simulink model "psb3phlinereclose"  (Simulink 6.0)
settings: Solver=FixedStepDiscrete  StartTime=0.0  StopTime=0.7  FixedStep=50e-6  RelTol=1e-4
InitFcn:
  | powericon('psbinitsys',bdroot);
undefined symbols (not defined in the file or in its folder): D1, Delta, rvar
libraries: powerlib2 x33, powerlib_extras x2
settings Model: Creator=sybille  LastModifiedBy=batserve  ExtModeTrigMode=oneshot  ExtModeArmWhenConnect=off  ExtModeAutoUpdateStatusClock=off
settings DataIOCC: LimitDataPoints=off  SignalLoggingName=sigsOut
settings OptimizationCC: BlockReduction=off  BooleanDataType=off
settings DebuggingCC: CheckExecutionContextPreStartOutputMsg=on  CheckExecutionContextRuntimeOutputMsg=on  SolverPrmCheckMsg=none
settings HardwareCC: TargetUnknown=on

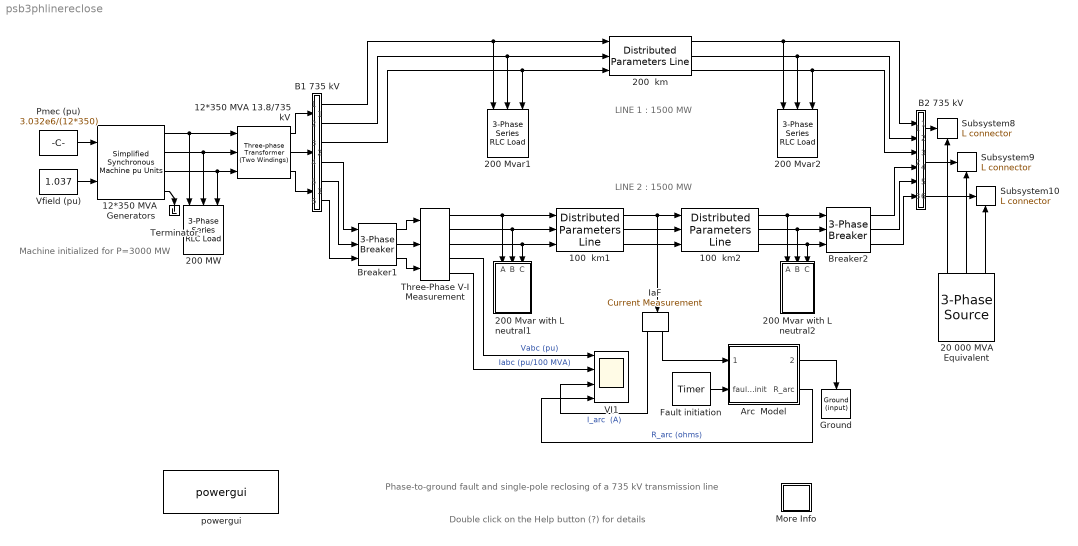
== system psb3phlinereclose ==
  note: Machine initialized
      |  for P=3000 MW
  note: Phase-to-ground fault and single-pole reclosing
      | of  a 735 kV transmission line
  note: Double click on the Help button (?) for details
  note: LINE 1 : 1500 MW
  note: LINE 2 : 1500 MW
  " Breaker1" : powerlib2/Elements/3-Phase Breaker  init_states=closed  sa=on  sb=off  sc=off  sw_times="[4/60  34/60]"  Ts=50e-6  comext=off  Ron=0.001  Rp=1e5  Cp=inf  mesure=None
  " Breaker2" : powerlib2/Elements/3-Phase Breaker  init_states=closed  sa=on  sb=off  sc=off  sw_times="[4/60  34/60]"  Ts=50e-6  comext=off  Ron=0.001  Rp=1e5  Cp=inf  mesure=None
  100  km1 : powerlib2/Elements/Distributed Parameters Line  Tag=PoWeRsYsTeMbLoCk  n=3  f=60  r=[0.01165 0.2676]  l="[0.8679e-3  3.008e-3]"  c="[13.41e-9  8.57e-9]"  lgt=100  x1=[0 -2.416e-007 4.728e+005 -5.555e+005;0.0001015 -2.421e-007 4.937e+005 -5.37e+005;0.0002031 -2.424e-007 5.139e+005 -5.177e+005;0.0003046 -2.422e-007 5.333e+005 -4.977e+005;0.0004062 -2.417e-007 5.52e+005 -4.769e+005;0.0005077 -2.408e-007 5.699e+005 -4.554e+005]  x2=[0 -1.471e-007 4.261e+005 -5.969e+005;0.0001015 -1.474e-007 4.486e+005 -5.801e+005;0.0002031 -1.474e-007 4.705e+005 -5.625e+005;0.0003046 -1.472e-007 4.917e+005 -5.441e+005;0.0004062 -1.468e-007 5.122e+005 -5.249e+005;0.0005077 -1.462e-007 5.319e+005 -5.049e+005]  x3=[0 -2.944e-010 398.8 -914.4;0.0001015 -2.663e-010 433.5 -898.5;0.0002031 -2.378e-010 467.6 -881.2;0.0003046 -2.089e-010 501 -862.7;0.0004062 -1.797e-010 533.6 -842.9;0.0005077 -1.503e-010 565.5 -821.9]  x4=[0 -3.362e-010 2831 -3827;0.0001015 -3.679e-010 2976 -3716;0.0002031 -3.99e-010 3116 -3599;0.0003046 -4.295e-010 3251 -3477;0.0004062 -4.594e-010 3382 -3350;0.0005077 -4.886e-010 3508 -3218]  x5=0.0005077  mesure=None  PSBOutputType=111111111111111111111111111111
  100  km2 : powerlib2/Elements/Distributed Parameters Line  Tag=PoWeRsYsTeMbLoCk  n=3  f=60  r=[0.01165 0.2676]  l="[0.8679e-3  3.008e-3]"  c="[13.41e-9  8.57e-9]"  lgt=100  x1=[0 -1.471e-007 4.261e+005 -5.969e+005;0.0001015 -1.474e-007 4.486e+005 -5.801e+005;0.0002031 -1.474e-007 4.705e+005 -5.625e+005;0.0003046 -1.472e-007 4.917e+005 -5.441e+005;0.0004062 -1.468e-007 5.122e+005 -5.249e+005;0.0005077 -1.462e-007 5.319e+005 -5.049e+005]  x2=[0 -4.673e-008 3.727e+005 -6.281e+005;0.0001015 -4.666e-008 3.965e+005 -6.134e+005;0.0002031 -4.652e-008 4.197e+005 -5.978e+005;0.0003046 -4.631e-008 4.422e+005 -5.813e+005;0.0004062 -4.604e-008 4.642e+005 -5.639e+005;0.0005077 -4.569e-008 4.854e+005 -5.457e+005]  x3=[0 -1.263e-010 506.9 -849.4;0.0001015 -9.531e-011 539.1 -829.3;0.0002031 -6.416e-011 570.4 -808.1;0.0003046 -3.291e-011 600.9 -785.7;0.0004062 -1.62e-012 630.6 -762.1;0.0005077 2.968e-011 659.3 -737.4]  x4=[0 -1.89e-010 2313 -4151;0.0001015 -2.214e-010 2470 -4059;0.0002031 -2.535e-010 2624 -3962;0.0003046 -2.852e-010 2773 -3859;0.0004062 -3.164e-010 2919 -3750;0.0005077 -3.472e-010 3060 -3635]  x5=0.0005077  mesure=None  PSBOutputType=111111111111111111111111111111
  12*350 MVA 13.8/735 kV : powerlib2/Elements/Three-phase Transformer (Two Windings)  Tag=PoWeRsYsTeMbLoCk  nominal=[ 12*350e6 , 60 ]  type1=Delta (D1)  params1=[ 13.8e3 , 0.002 , 0.08 ]  type2=Yg  params2=[ 735e3 , 0.002 , 0.08 ]  ynsat=off  rmag=500  lm=500  sat=[ 0,0 ; 0.0024,1.2 ; 1.0,1.52 ]  hyst=off  matfile='hysteresis'  sif=off  phi0=[ 0.8 , -0.8 , 0.7 ]  initialslopes=[+1 +1 +1]  mesure=None  PSBOutputType=111
  12*350 MVA  Generators : powerlib2/Machines/Simplified Synchronous  Machine  pu Units  Tag=PoWeRsYsTeMbLoCk  conType=3-wire Y  x1=[ 12*350e6,13.8e3,60 ]  x2=[ inf,0,2 ]  x3=[ 0.22/15, 0.22 ]  x4=[0 2.57573 0.717405 0.717405 0.717405 -11.4304 -131.43 108.57]  PSBOutputType=1110  iounits=0  LoadFlowParameters=[1 3000000000 0 0 0]
  20 000 MVA Equivalent : powerlib2/Electrical Sources/3-Phase Source  Tag=PoWeRsYsTeMbLoCk  Orientation=up  V=735e3  Phi=0  F=60  InternalConnection=Yg  RLoff=on  R=735^2/20000/10  L=735^2/20000/377  Psc=20000e6  Vbase=735e3  XRratio=10  PSBOutputType=111
  200  km : powerlib2/Elements/Distributed Parameters Line  Tag=PoWeRsYsTeMbLoCk  n=3  f=60  r=[0.01165 0.2676]  l="[0.8679e-3  3.008e-3]"  c="[13.41e-9  8.57e-9]"  lgt=200  x1=[0 -2.332e-007 3.976e+005 -6.116e+005;0.0002031 -2.374e-007 4.433e+005 -5.794e+005;0.0004062 -2.403e-007 4.863e+005 -5.438e+005;0.0006093 -2.417e-007 5.264e+005 -5.05e+005;0.0008124 -2.417e-007 5.635e+005 -4.632e+005;0.001015 -2.403e-007 5.973e+005 -4.188e+005]  x2=[0 -4.613e-008 2.891e+005 -6.707e+005;0.0002031 -4.657e-008 3.395e+005 -6.466e+005;0.0004062 -4.675e-008 3.88e+005 -6.188e+005;0.0006093 -4.665e-008 4.342e+005 -5.873e+005;0.0008124 -4.628e-008 4.779e+005 -5.524e+005;0.001015 -4.563e-008 5.187e+005 -5.142e+005]  x3=[0 -4.038e-010 276 -953;0.0002031 -3.531e-010 348.1 -929.1;0.0004062 -3.004e-010 418.1 -899.7;0.0006093 -2.46e-010 485.7 -865.1;0.0008124 -1.901e-010 550.5 -825.4;0.001015 -1.331e-010 612 -780.9]  x4=[0 -1.229e-011 1756 -4400;0.0002031 -7.699e-011 2087 -4253;0.0004062 -1.412e-010 2407 -4081;0.0006093 -2.046e-010 2712 -3885;0.0008124 -2.669e-010 3001 -3666;0.001015 -3.275e-010 3273 -3426]  x5=0.001015  mesure=None  PSBOutputType=111111111111111111111111111111
  200 MW : powerlib2/Elements/3-Phase Series RLC Load  Orientation=down  Vpp=13.8e3  fn=60  P3=200e6  QL3=0  QC3=0
  200 Mvar with L neutral1 : Subsystem  Orientation=down
  200 Mvar with L neutral2 : Subsystem  Orientation=down
  200 Mvar1 : powerlib2/Elements/3-Phase Series RLC Load  Orientation=down  Vpp=735e3  fn=60  P3=200e6/250  QL3=200e6  QC3=0
  200 Mvar2 : powerlib2/Elements/3-Phase Series RLC Load  Orientation=down  Vpp=735e3  fn=60  P3=200e6/250  QL3=200e6  QC3=0
  Arc  Model : Subsystem  mask(Arc model){Rarc_var=on, Rarc_fixed=0.1, Rparam=[56.54 0.006375], I0=50, Ts=50e-6}
      mask prompts: Rarc_var "Variable arc resistance :"; Rarc_fixed "Arc resistance for fixed arc resistance :"; Rparam "Arc parameters for variable arc resistance [Ro k] : :"; I0 "Current threshold for arc extinction Io (A rms) :"; Ts "Sample time (s) :"
      mask help:
      | This block implements a variable or fixed arc resistance model.
      |
      | Input 1, output 1:  Connection terminals of the arc
      |                              resistance.
      | Input 2 :    Control signal for the fault initiation
      | Use a short pulse of 1 cycle. Once fault current starts flowing, it is sustained by the arc ionized path.
      | Output 2:  Arc resitance
      |
      | If you check the 'Variable arc resistance' box, the mean arc resistance will be a function of the arc current, according to equation. Otherwise, the resistance will be kept constant.
      |
      |        Rarc= Ro*exp(-k*i)
      |
      | where:   i = rms value of the arc current (A)
      |              Ro, k = arc parameters
      |
      | The arc extinguishes at the next zero current crossing after its  rms value has fallen  below  the specified threshold current Io.
      mask init:
      | if strcmp(Rarc_var,'on'), rvar=1; else, rvar=0; end
      | R0=Rparam(1);
      | k=Rparam(2);
  B1 735 kV : Subsystem
      mask Display: disp('')
  B2 735 kV : Subsystem
      mask Display: disp('')
  Fault initiation : powerlib_extras/Control  Blocks/Timer  t=[ 1/60 2/60 ]  e="[1 0  ]"
  Ground : powerlib2/Connectors/Ground (input)  Tag=PoWeRsYsTeMbLoCk  Orientation=down
  IaF : powerlib2/Measurements/Current Measurement  Tag=PoWeRsYsTeMmEaSuReMeNt  Orientation=down  PhasorSimulation=off  OutputType=Magnitude  PSBOutputType=01  PSBequivalent=0
  More Info : Subsystem
      mask Display: disp('?')
  Pmec (pu) : Constant  Value=3.032e6/(12*350)
  Subsystem10 : powerlib2/Connectors/L connector  Tag=PoWeRsYsTeMbLoCk  Orientation=up
  Subsystem8 : powerlib2/Connectors/L connector  Tag=PoWeRsYsTeMbLoCk  Orientation=up
  Subsystem9 : powerlib2/Connectors/L connector  Tag=PoWeRsYsTeMbLoCk  Orientation=up
  Terminator : Terminator
      settings: Orientation=down
  Three-Phase V-I Measurement : powerlib2/Measurements/Three-Phase V-I Measurement  Tag=PoWeRsYsTeMmEaSuReMeNt  VChoice=phase-to-ground  ualv=off  labelV=V1  Vpu=on  Vbase=735e3  IChoice=yes  ualc=off  labelC=I1  Ppu=on  Pbase=100e6  OutputType=Magnitude  PhasorSimulation=off  PSBequivalent=1  PSBOutputType=11100
  VI1 : Scope  NumInputPorts=4
      settings: TimeRange=0.7000000000000001  YMin=-2~-100~-50000~0  YMax=2~100~50000~100  DataFormat=Array
  Vfield (pu) : Constant  Value=1.037
  powergui : powerlib2/powergui  Frange=logspace(0,3,50)  Ylog=off  Xlog=off  save=off  variable=ZData  ZoomFFT=on  StartTime=0.0  cycles=1  DisplayStyle=off  fundamental=60  FreqAxis=off  MaxFrequency=1000  frequencyindice=60  frequencyindicesteady=1  RmsSteady=1  display=off  Ts=50e-6  methode=off  frequency=60  echomessages=off
  wires:
  " Breaker1"/1 -> Three-Phase V-I Measurement/1
  " Breaker1"/2 -> Three-Phase V-I Measurement/2
  " Breaker1"/3 -> Three-Phase V-I Measurement/3
  12*350 MVA 13.8/735 kV/1 -> B1 735 kV/1(A1)
  12*350 MVA 13.8/735 kV/2 -> B1 735 kV/2(B1)
  12*350 MVA 13.8/735 kV/3 -> B1 735 kV/3(C1)
  B1 735 kV/4(A4) -> " Breaker1"/1
  B1 735 kV/5(B4) -> " Breaker1"/2
  B1 735 kV/6(C4) -> " Breaker1"/3
  12*350 MVA  Generators/1 -> 12*350 MVA 13.8/735 kV/1, 200 MW/1
  12*350 MVA  Generators/2 -> 12*350 MVA 13.8/735 kV/2, 200 MW/2
  12*350 MVA  Generators/3 -> 12*350 MVA 13.8/735 kV/3, 200 MW/3
  Vfield (pu)/1 -> 12*350 MVA  Generators/2
  Pmec (pu)/1 -> 12*350 MVA  Generators/1
  " Breaker2"/3 -> B2 735 kV/6(C2)
  B2 735 kV/1(A3) -> Subsystem8/Enable
  20 000 MVA Equivalent/1 -> Subsystem8/1
  B2 735 kV/2(B3) -> Subsystem9/Enable
  20 000 MVA Equivalent/2 -> Subsystem9/1
  B2 735 kV/3(C3) -> Subsystem10/Enable
  20 000 MVA Equivalent/3 -> Subsystem10/1
  " Breaker2"/1 -> B2 735 kV/4(A2)
  " Breaker2"/2 -> B2 735 kV/5(B2)
  100  km2/1 -> " Breaker2"/1, 200 Mvar with L neutral2/1(A)
  100  km2/2 -> " Breaker2"/2, 200 Mvar with L neutral2/2(B)
  100  km2/3 -> " Breaker2"/3, 200 Mvar with L neutral2/3(C)
  100  km1/1 -> 100  km2/1, IaF/1
  B1 735 kV/1(A3) -> 200  km/1, 200 Mvar1/1
  B1 735 kV/2(B3) -> 200  km/2, 200 Mvar1/2
  B1 735 kV/3(C3) -> 200  km/3, 200 Mvar1/3
  200  km/1 -> B2 735 kV/1(A1`), 200 Mvar2/1
  200  km/2 -> B2 735 kV/2(B1), 200 Mvar2/2
  200  km/3 -> B2 735 kV/3(C1), 200 Mvar2/3
  Three-Phase V-I Measurement/1 -> 100  km1/1, 200 Mvar with L neutral1/1(A)
  Three-Phase V-I Measurement/2 -> 100  km1/2, 200 Mvar with L neutral1/2(B)
  Three-Phase V-I Measurement/3 -> 100  km1/3, 200 Mvar with L neutral1/3(C)
  100  km1/3 -> 100  km2/3
  100  km1/2 -> 100  km2/2
  Three-Phase V-I Measurement/4 -> VI1/1  "Vabc (pu)"
  Fault initiation/1 -> Arc  Model/2(fault_init)
  Arc  Model/1(2) -> Ground/1
  IaF/2 -> Arc  Model/1(1)
  IaF/1 -> VI1/3  "I_arc  (A)"
  Arc  Model/2(R_arc) -> VI1/4  "R_arc (ohms)"
  Three-Phase V-I Measurement/5 -> VI1/2  "Iabc (pu/100 MVA)"
  12*350 MVA  Generators/4 -> Terminator/1

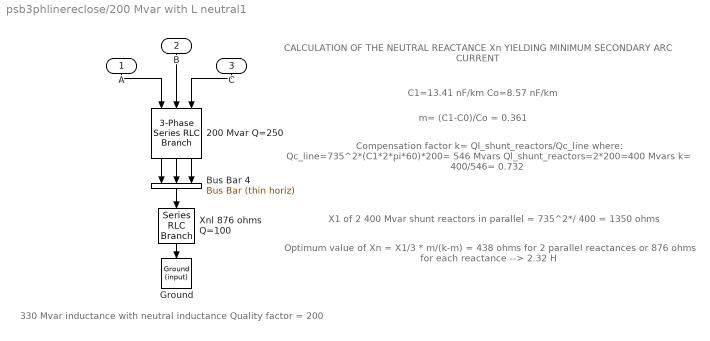
== system psb3phlinereclose/200 Mvar with L neutral1 ==
  note: CALCULATION OF THE NEUTRAL REACTANCE Xn
      | YIELDING MINIMUM SECONDARY ARC CURRENT
  note: X1 of 2 400 Mvar shunt reactors in parallel = 735^2*/ 400 = 1350 ohms
  note: Optimum value of Xn = X1/3 * m/(k-m) = 438 ohms for 2 parallel reactances
      | or 876 ohms for each reactance --> 2.32 H
  note: Compensation factor k= Ql_shunt_reactors/Qc_line
      | where:
      |  Qc_line=735^2*(C1*2*pi*60)*200= 546 Mvars
      |  Ql_shunt_reactors=2*200=400 Mvars
      | k= 400/546= 0.732
  note: m= (C1-C0)/Co = 0.361
  note: C1=13.41 nF/km Co=8.57 nF/km
  note: 330 Mvar inductance
      | with neutral inductance
      | Quality factor = 200
  A : Inport  Orientation=down  Port=1  LatchInput=off
  B : Inport  Orientation=down  Port=2  LatchInput=off
  C : Inport  Orientation=down  Port=3  LatchInput=off
  200 Mvar Q=250 : powerlib2/Elements/3-Phase Series RLC Branch   Orientation=down  R=735^2/200/250  L=735^2/200/377  C=inf
  Bus Bar 4 : powerlib2/Connectors/Bus Bar (thin horiz)  Tag=PoWeRsYsTeMbLoCk  Orientation=down  input=3  output=1  PSBOutputType=111111111111111111111111111111111111111111111111111111111111111111111111111111111111
  Ground : powerlib2/Connectors/Ground (input)  Tag=PoWeRsYsTeMbLoCk  Orientation=down
  Xnl 876 ohms Q=100 : powerlib2/Elements/Series RLC Branch  Tag=PoWeRsYsTeMbLoCk  Orientation=down  a=876/100  b=876/377  c=inf  mesure=None  PSBOutputType=1
  wires:
  A/1 -> 200 Mvar Q=250/1
  B/1 -> 200 Mvar Q=250/2
  C/1 -> 200 Mvar Q=250/3
  200 Mvar Q=250/1 -> Bus Bar 4/1
  200 Mvar Q=250/3 -> Bus Bar 4/3
  200 Mvar Q=250/2 -> Bus Bar 4/2
  Bus Bar 4/1 -> Xnl 876 ohms Q=100/1
  Xnl 876 ohms Q=100/1 -> Ground/1

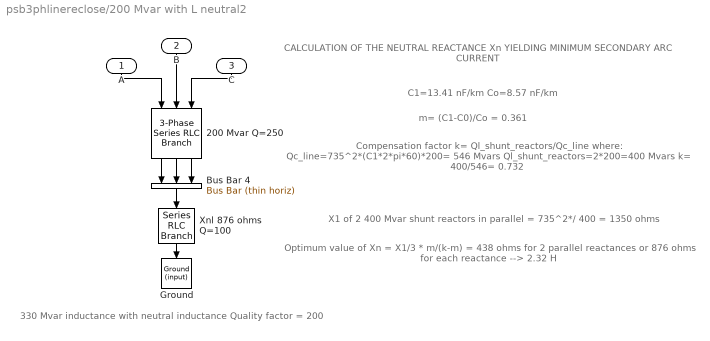
== system psb3phlinereclose/200 Mvar with L neutral2 ==
  note: 330 Mvar inductance
      | with neutral inductance
      | Quality factor = 200
  note: C1=13.41 nF/km Co=8.57 nF/km
  note: m= (C1-C0)/Co = 0.361
  note: Compensation factor k= Ql_shunt_reactors/Qc_line
      | where:
      |  Qc_line=735^2*(C1*2*pi*60)*200= 546 Mvars
      |  Ql_shunt_reactors=2*200=400 Mvars
      | k= 400/546= 0.732
  note: Optimum value of Xn = X1/3 * m/(k-m) = 438 ohms for 2 parallel reactances
      | or 876 ohms for each reactance --> 2.32 H
  note: X1 of 2 400 Mvar shunt reactors in parallel = 735^2*/ 400 = 1350 ohms
  note: CALCULATION OF THE NEUTRAL REACTANCE Xn
      | YIELDING MINIMUM SECONDARY ARC CURRENT
  A : Inport  Orientation=down  Port=1  LatchInput=off
  B : Inport  Orientation=down  Port=2  LatchInput=off
  C : Inport  Orientation=down  Port=3  LatchInput=off
  200 Mvar Q=250 : powerlib2/Elements/3-Phase Series RLC Branch   Orientation=down  R=735^2/200/250  L=735^2/200/377  C=inf
  Bus Bar 4 : powerlib2/Connectors/Bus Bar (thin horiz)  Tag=PoWeRsYsTeMbLoCk  Orientation=down  input=3  output=1  PSBOutputType=111111111111111111111111111111111111111111111111111111111111111111111111111111111111
  Ground : powerlib2/Connectors/Ground (input)  Tag=PoWeRsYsTeMbLoCk  Orientation=down
  Xnl 876 ohms Q=100 : powerlib2/Elements/Series RLC Branch  Tag=PoWeRsYsTeMbLoCk  Orientation=down  a=876/100  b=876/377  c=inf  mesure=None  PSBOutputType=1
  wires:
  Xnl 876 ohms Q=100/1 -> Ground/1
  Bus Bar 4/1 -> Xnl 876 ohms Q=100/1
  200 Mvar Q=250/2 -> Bus Bar 4/2
  200 Mvar Q=250/3 -> Bus Bar 4/3
  200 Mvar Q=250/1 -> Bus Bar 4/1
  C/1 -> 200 Mvar Q=250/3
  B/1 -> 200 Mvar Q=250/2
  A/1 -> 200 Mvar Q=250/1

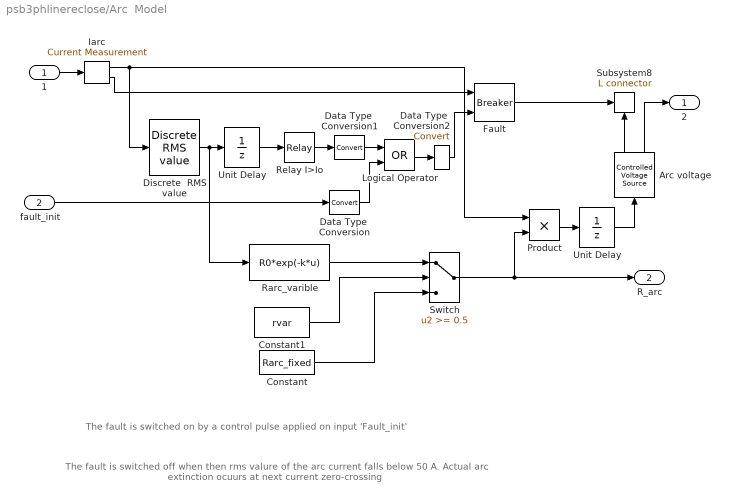
== system psb3phlinereclose/Arc  Model ==
  note: The fault is switched on by a control pulse applied on input 'Fault_init'
  note: The fault is switched off when then rms valure of the arc current falls below  50 A.
      | Actual arc extinction ocuurs at next current zero-crossing
  1 : Inport  Port=1  LatchInput=off
  fault_init : Inport  Port=2  LatchInput=off
  Arc voltage : powerlib2/Electrical Sources/Controlled Voltage Source  Tag=PoWeRsYsTeMbLoCk  Description=source block  Orientation=up  initsrc=on  srctyp=AC  iv=0  iph=0  ifreq=0  mesure=None  PSBOutputType=11
  Constant : Constant  Value=Rarc_fixed
  Constant1 : Constant  Value=rvar
  Data Type  Conversion : DataTypeConversion  OutDataTypeMode=boolean  SaturateOnIntegerOverflow=on  RndMeth=Zero
  Data Type  Conversion1 : DataTypeConversion  OutDataTypeMode=boolean  SaturateOnIntegerOverflow=on  RndMeth=Zero
  Data Type  Conversion2 : DataTypeConversion  OutDataTypeMode=double  SaturateOnIntegerOverflow=on  RndMeth=Zero
  Discrete  RMS value : powerlib_extras/Discrete Measurements/Discrete  RMS value  Freq=60  Mag_Init=0  Ts=Ts
  Fault : powerlib2/Elements/Breaker  Tag=PoWeRsYsTeMbLoCk  a=.001  c=0  rs=inf  cs=0  times="[ 4/60  5/60 ]"  Ts=0  comext=on  mesure=None  PSBOutputType=1
  Iarc : powerlib2/Measurements/Current Measurement  Tag=PoWeRsYsTeMmEaSuReMeNt  PhasorSimulation=off  OutputType=Magnitude  PSBOutputType=01  PSBequivalent=0
  Logical Operator : Logic  Operator=OR
  Product : Product  SaturateOnIntegerOverflow=on  InputSameDT=on
  Rarc_varible : Fcn  Expr=R0*exp(-k*u)
  Relay I>Io : Relay  OnSwitchValue=I0*1.2  OffSwitchValue=I0  ZeroCross=off
  Subsystem8 : powerlib2/Connectors/L connector  Tag=PoWeRsYsTeMbLoCk  Orientation=up
  Switch : Switch  Threshold=0.5  ZeroCross=off  InputSameDT=on
  Unit Delay : UnitDelay  SampleTime=Ts
  "Unit Delay " : UnitDelay  SampleTime=Ts
  2 : Outport
  R_arc : Outport  Port=2
  wires:
  1/1 -> Iarc/1
  Fault/1 -> Subsystem8/Enable
  Iarc/2 -> Fault/1
  Iarc/1 -> Discrete  RMS value/1, Product/1
  Discrete  RMS value/1 -> "Unit Delay "/1, Rarc_varible/1
  Rarc_varible/1 -> Switch/1
  Switch/1 -> Product/2, R_arc/1
  Constant/1 -> Switch/3
  Constant1/1 -> Switch/2
  Arc voltage/1 -> Subsystem8/1
  Arc voltage/2 -> 2/1
  Product/1 -> Unit Delay/1
  Unit Delay/1 -> Arc voltage/1
  "Unit Delay "/1 -> Relay I>Io/1
  fault_init/1 -> Data Type  Conversion/1
  Data Type  Conversion/1 -> Logical Operator/2
  Relay I>Io/1 -> Data Type  Conversion1/1
  Data Type  Conversion1/1 -> Logical Operator/1
  Logical Operator/1 -> Data Type  Conversion2/1
  Data Type  Conversion2/1 -> Fault/2

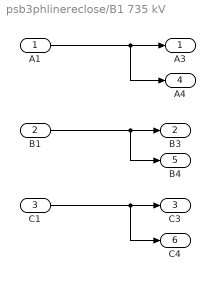
== system psb3phlinereclose/B1 735 kV ==
  A1 : Inport  Port=1  LatchInput=off
  B1 : Inport  Port=2  LatchInput=off
  C1 : Inport  Port=3  LatchInput=off
  A3 : Outport  InitialOutput=0
  B3 : Outport  Port=2  InitialOutput=0
  C3 : Outport  Port=3  InitialOutput=0
  A4 : Outport  Port=4  InitialOutput=0
  B4 : Outport  Port=5  InitialOutput=0
  C4 : Outport  Port=6  InitialOutput=0
  wires:
  C1/1 -> C3/1, C4/1
  B1/1 -> B3/1, B4/1
  A1/1 -> A3/1, A4/1

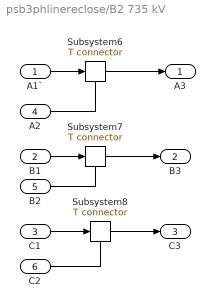
== system psb3phlinereclose/B2 735 kV ==
  A1` : Inport  Port=1  LatchInput=off
  B1 : Inport  Port=2  LatchInput=off
  C1 : Inport  Port=3  LatchInput=off
  A2 : Inport  Port=4  LatchInput=off
  B2 : Inport  Port=5  LatchInput=off
  C2 : Inport  Port=6  LatchInput=off
  Subsystem6 : powerlib2/Connectors/T connector  Tag=PoWeRsYsTeMbLoCk  PSBOutputType=1
  Subsystem7 : powerlib2/Connectors/T connector  Tag=PoWeRsYsTeMbLoCk  PSBOutputType=1
  Subsystem8 : powerlib2/Connectors/T connector  Tag=PoWeRsYsTeMbLoCk  PSBOutputType=1
  A3 : Outport  InitialOutput=0
  B3 : Outport  Port=2  InitialOutput=0
  C3 : Outport  Port=3  InitialOutput=0
  wires:
  C2/1 -> Subsystem8/Enable
  A2/1 -> Subsystem6/Enable
  B2/1 -> Subsystem7/Enable
  B1/1 -> Subsystem7/1
  C1/1 -> Subsystem8/1
  A1`/1 -> Subsystem6/1
  Subsystem8/1 -> C3/1
  Subsystem7/1 -> B3/1
  Subsystem6/1 -> A3/1

== system psb3phlinereclose/More Info ==
  note: Choose  Simulation/Start and observe the voltage and current waveforms on the 4-trace oscilloscope.
      |
      | Observe the three phase-to-ground voltages and currents at sending end of line 2, and the current flowing into the fault.The line voltages
      | and currents are measured with the 3-phase measurement bus of the Extra library. It allows to output voltages and currents directly in pu.
      | The machine has been previously initialized to deliver 3000 MW of power at 1 pu voltage. (with  the Load Flow option of the Powergui)
      | The line currents flowing into each line are therefore 15pu/100 MVA as observed on trace 2.
      |
      | The fault current (I_arc) is measured in amperes. It reaches 22 kA during the first cycle, then it drops to a very small value  after 3 cycles
      |  when the two line breakers open. Use Y-zoom to look at the secondary arc current. It contains a slowly  decaying DC component and a
      |  fundamental component (12 A peak) . As its rms value is below 50 A, the arc extinguishes at the first current zero crossing.
      |
      | Now, open the Arc Model block menu and change the arc model to a fixed resistance (0.1 ohm).
      | Restart the simulation. You will notice that the DC component of the arc current prevents arc extinction, so that the line is now  reclosed on a fault.
      | You can also suppress the neutral reactance in the two shunt reactance blocks and see the impact on the secondary arc current.
  note: Demonstration
  note: Two 735 kV parallel lines, 200 km long, transmit 3000 MW of power from a generation plant (12 generators of 350 MVA) to
      | to an equivalent network having a short circuit level of 20 GVA.
      |
      | The generation plant is simulated with a simplified synchronous machine  (subtransient reactance of 0.22 pu).
      | The machine is connected to the transmission network through a 13.8 kV/ 735 kV Wye-Delta transformer.
      |
      | The line models are distributed parameter lines. The lines are assumed to be transposed and their parameters R,L,C /km are specified
      | in positive- and zero-sequence components. Each line is shunt compensated by two shunt reactors of 200 Mvars each, connected at line ends.
      | Applying single pole reclosing at this voltage level is made possible by the use of neutral inductances for the two shunt reactances of line 2.
      | Otherwise, the 'secondary arc current'  which is induced into the fault ( mainly because of the capacitive coupling between the two sound phases
      | and the faulted phase) would be too high to allow arc extinction after opening of  line breakers on the faulted phase.
      | If you open the two shunt reactance blocks of line 2, you will  see how the optimum neutral inductance is calculated.
  note: This demonstration ilustrates the use of three-phase blocks
      | to study of a single-pole reclosing on  a 735-kV transmission line
  note: Circuit Description
  note: A  phase-to-ground fault is applied at the middle of line 2. In order to apply the fault along the line,
      | this line  is simulated in two sections of 100 km. As soon as the fault is detected by the protection relays (not simulated here) ,
      | an opening command is sent to the two line breakers of the faulted phase. The breaker are kept open during a certain 'dead time' ,
      | usually around 0.5 s, during which the arc normally  extinguishes, then the two breakers are reclosed
      | .
      | When the two line breakers are tripped on the faulted phase, the fault current is interrupted but a small current will continue  to flow through the arc.
      | If this  secondary arc current  is too large (typically above 50 A) , the arc cannot extinguish and the breaker will reclose on the fault..
  note: Fault and line switching
  note: The arc is modelled by a fixed or non-linear resistance R = f(Iarc_rms). The arc extinguishes when its rms current falls below a
      | certain threshold value (typically 50 A) defined in the arc model block. Open the Arc Model block and look at the arc parameters.
      | The mean arc resistance  is programmed as an exponential function of the rms current. The mean arc resistance increases when the rms arc current decreases
      | so that the time for arc current to decay below the threshold value is shortened . (With the specified parameters, Rarc = 0.1ohm and 30 ohms respectively
      | for currents of 1kA and 100A). The Arc Model block  is a masked block. Use 'Look under mask' to see how the arc model is implemented.
      |
      | Open the blocks simulating the two line breakers. See how the line opening/reclosing sequence is programmed.
      | The fault is applied at t = 1 cycle. Then, the opening command is sent to both breakers  at t = 4 cycles (3 cycles detection+ opening time).
      | The two breakers are reclosed at t = 34 cycles after a dead time of 30 cycles, during which the arc creating the fault should extinguish.
  note: Arc model
  note: G. Sybille (Hydro-Quebec)
